simulink model "final"  (R2020b)
settings: Solver=VariableStepAuto  StartTime=0.0  StopTime=16  RelTol=1e-3
values from neighbouring files (symbols this model uses):
  a = 0.0032    [parametros.m]
  c = 1*10^(3.5)    (= 3162.27766017)    [parametros.m]
  k = 2e6    (= 2000000)    [parametros.m]
  K = K3    [parametros.m]
  m = 2000    [parametros.m]
  T = 0.001    [parametros.m]
undefined symbols (not defined in the file or in its folder): DiscIntNeverNeededParam, L, sigbuilder_block
libraries: commchan3 x1, mcbcontrolslib x1, simulink_extras x1, robotcorelib x1, simulink x1
settings Model: Creator=tinsu  LastModifiedBy=tinsu

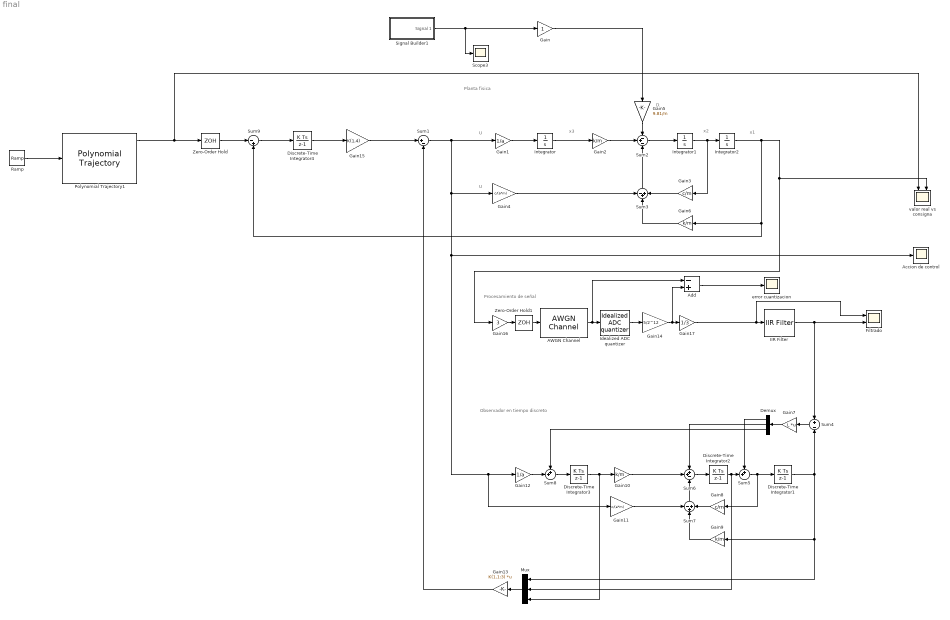
== system final ==
  note: D
  note: Procesamiento de señal
  note: x1
  note: x2
  note: x3
  note: Planta fisica
  note: Observador en tiempo discreto
  note: U
  note: U
  AWGN Channel : commchan3/AWGN Channel  InputProcessing=Columns as channels (frame based)  seed=99  noiseMode="Signal to noise ratio  (SNR)"  EbNodB=10  EsNodB=10  SNRdB=82  bitsPerSym=1  Ps=1  Tsym=1  variance=1
  Accion de control : Scope
  Add : Sum  Inputs=-+
  Demux : Demux  Outputs=3
  Discrete-Time Integrator{1..4} (4 alike) : DiscreteIntegrator  SampleTime=T  ICPrevOutput=DiscIntNeverNeededParam  ICPrevScaledInput=DiscIntNeverNeededParam
  Filtrado : Scope  NumInputPorts=2
  Gain : Gain
  Gain1 : Gain  Gain=1/a
  Gain{2,6,9..10} (4 alike) : Gain  Gain=k/m
  Gain11 : Gain  Gain=c/(a*m)
  Gain12 : Gain  Gain=1/a
  Gain13 : Gain  Gain=K(1,1:3)  Multiplication=Matrix(K*u) (u vector)
  Gain14 : Gain  Gain=5/2^12
  Gain15 : Gain  Gain=K(1,4)
  Gain16 : Gain  Gain=3
  Gain17 : Gain  Gain=1/3
  Gain3 : Gain  Gain=c/m
  Gain4 : Gain  Gain=c/(a*m)
  Gain5 : Gain  Gain=9.81/m
  Gain7 : Gain  Gain=L  Multiplication=Matrix(K*u)
  Gain8 : Gain  Gain=c/m
  IIR Filter : mcbcontrolslib/IIR Filter  Filter_constant=.28
      settings: SourceProductBaseCode=MT
  Idealized ADC quantizer : simulink_extras/Additional Discrete/Idealized ADC quantizer  NumberOfConverterBits=12  Vmin=0  Vmax=5  OutputDataType=double  OutputNegativeValues=off
  Integrator : Integrator
  Integrator1 : Integrator
  Integrator2 : Integrator
  Mux : Mux  Inputs=3
  Polynomial Trajectory1 : robotcorelib/Polynomial Trajectory  WaypointSource=Internal  Waypoints=[ 0, 1.5, 1.5,1]  TimePoints=[ 2, 6, 7, 10]  TimeInterval=[ 1, 4 ]  Method=Cubic Polynomial  ParameterSource=Internal  VelocityBoundaryCondition=zeros( 1, 4 )  AccelerationBoundaryCondition=zeros( 2, 5 )  SimulateUsing=Interpreted execution
  Ramp : simulink/Sources/Ramp  slope=1  start=0  InitialOutput=0
  Scope3 : Scope
  Signal Builder1 : Subsystem  Tag=STV Subsys  LoadFcn=sigbuilder_block('load');  StartFcn=sigbuilder_block('start');  StopFcn=sigbuilder_block('stop');  ClipboardFcn=sigbuilder_block('clipboard');  mask(Sigbuilder block){tuvar=[0:10]}
      mask help: Simulink:masks:SigbuilderBlock_MD
      mask init:
      | if ~strcmp(get_param(bdroot(gcbh),'SimulationStatus'),'stopped') tuvar = sigbuilder_block('maskInit'); end
      settings: CopyFcn=sigbuilder_block('copy');  DeleteFcn=sigbuilder_block('delete');  ModelCloseFcn=sigbuilder_block('modelClose');  PreSaveFcn=sigbuilder_block('preSave');  PauseFcn=sigbuilder_block('pause');  ContinueFcn=sigbuilder_block('continue');  NameChangeFcn=sigbuilder_block('namechange');  OpenFcn=sigbuilder_block('open',[437.6 153 550.4 359.25 ]);  CloseFcn=sigbuilder_block('close');
      mask Display: plot(0, 0, 100, 100,[2, 2, 32, 32, 2], [68, 8, 8, 68, 68],[32, 2], [38, 38], [32, 19, 2],[53, 60, 44], [32, 17, 17, 2],[16, 16, 31, 31]);txt = getActiveGroup(gcbh);text(2, 100, txt,'verticalAlignment', 'top');
  Sum1 : Sum  Inputs=|+-
  Sum2 : Sum  Inputs=-+-
  Sum3 : Sum  Inputs=-++
  Sum4 : Sum  Inputs=+-
  Sum5 : Sum  Inputs=++|
  Sum6 : Sum  Inputs=++-
  Sum7 : Sum  Inputs=-++
  Sum8 : Sum  Inputs=++|
  Sum9 : Sum  Inputs=|-+
  Zero-Order Hold : ZeroOrderHold  SampleTime=T
  Zero-Order Hold1 : ZeroOrderHold  SampleTime=T
  error cuantizacion : Scope
  valor real vs consigna : Scope  NumInputPorts=2
  wires:
  Sum1/1 -> Gain1/1, Accion de control/1, Gain12/1, Gain11/1, Gain4/1
  Gain1/1 -> Integrator/1
  Integrator/1 -> Gain2/1
  Gain2/1 -> Sum2/2
  Sum2/1 -> Integrator1/1
  Gain3/1 -> Sum3/3
  Sum3/1 -> Sum2/3
  Gain4/1 -> Sum3/1
  Gain5/1 -> Sum2/1
  Integrator1/1 -> Gain3/1, Integrator2/1
  Gain6/1 -> Sum3/2
  Sum4/1 -> Gain7/1
  Gain7/1 -> Demux/1
  Sum5/1 -> Discrete-Time Integrator1/1, Gain8/1
  Demux/1 -> Sum5/1
  Discrete-Time Integrator2/1 -> Mux/2, Sum5/2
  Sum6/1 -> Discrete-Time Integrator2/1
  Demux/2 -> Sum6/1
  Discrete-Time Integrator1/1 -> Gain9/1, Mux/1, Sum4/2
  Gain8/1 -> Sum7/3
  Gain9/1 -> Sum7/2
  Discrete-Time Integrator3/1 -> Gain10/1, Mux/3
  Gain11/1 -> Sum7/1
  Sum8/1 -> Discrete-Time Integrator3/1
  Gain12/1 -> Sum8/2
  Demux/3 -> Sum8/1
  Mux/1 -> Gain13/1
  Gain13/1 -> Sum1/2
  Gain10/1 -> Sum6/2
  Ramp/1 -> Polynomial Trajectory1/1
  Zero-Order Hold/1 -> Sum9/1
  IIR Filter/1 -> Sum4/1, Filtrado/2
  Integrator2/1 -> Gain16/1, valor real vs consigna/2, Gain6/1, Sum9/2
  Idealized ADC quantizer/1 -> Gain14/1
  Gain14/1 -> Add/2, Gain17/1
  AWGN Channel/1 -> Add/1, Idealized ADC quantizer/1
  Zero-Order Hold1/1 -> AWGN Channel/1
  Gain16/1 -> Zero-Order Hold1/1
  Gain17/1 -> Filtrado/1, IIR Filter/1
  Add/1 -> error cuantizacion/1
  Polynomial Trajectory1/1 -> valor real vs consigna/1, Zero-Order Hold/1
  Discrete-Time Integrator4/1 -> Gain15/1
  Sum9/1 -> Discrete-Time Integrator4/1
  Gain15/1 -> Sum1/1
  Signal Builder1/1(Signal 1) -> Scope3/1, Gain/1
  Gain/1 -> Gain5/1
  Sum7/1 -> Sum6/3

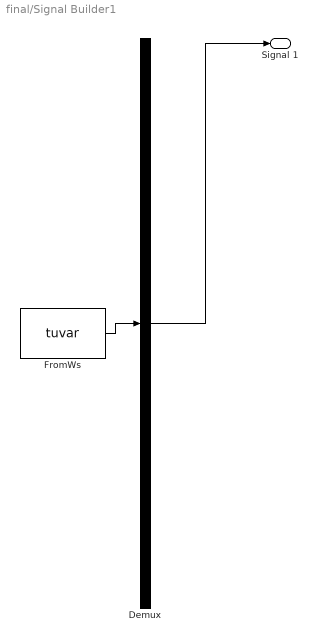
== system final/Signal Builder1 ==
  Demux : Demux  Tag=STV Demux  Outputs=1
      settings: DisplayOption=none
  FromWs : FromWorkspace  Tag=STV FromWs  VariableName=tuvar
      SigBuilderData=|
      | common.afterFinalStr = 'Extrapolate'
      | common.sampleTime = 0
      | dataSet.timeRange = [0 20]
      | dataSet.name = 'Group 1'
      | sbobj.Groups.Name = 'Group 1'
      | sbobj.Groups.Signals.Name = 'Signal 1'
      | sbobj.Groups.Signals.XData = [0 12 12 15 15 20]
      | sbobj.Groups.Signals.YData = [0 0 700 700 0 0]
      | sbobj.Groups.TimeRange = [0 20]
  Signal 1 : Outport  Tag=STV Outport
  wires:
  Demux/1 -> Signal 1/1
  FromWs/1 -> Demux/1
